simulink model "cgMassInertia"  (R2024a)
settings: configuration reference "autoCodeSILConfigurationParams" (kept outside this file)
undefined symbols (not defined in the file): stepSize_s, vehicleParams
settings Model: Creator=GTAR  LastModifiedBy=jerem
settings ConfigSetRef: SourceName=autoCodeSILConfigurationParams  SourceLocation=Base Workspace

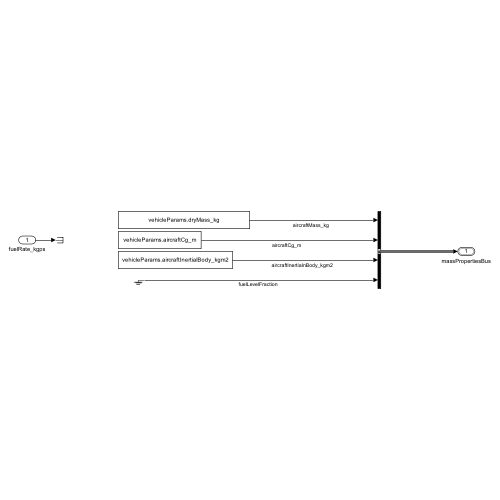
[thumbnail: Simulink's stored preview of the top-level diagram]
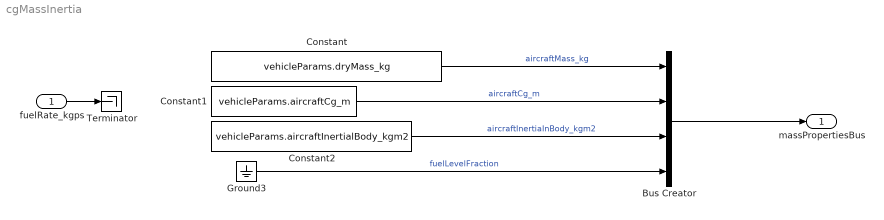
== system cgMassInertia ==
  fuelRate_kgps : Inport
  Bus Creator : BusCreator  Inputs=4  OutDataTypeStr=Bus: MassPropertiesBus  NonVirtualBus=on
  Constant : Constant  Value=vehicleParams.dryMass_kg  SampleTime=stepSize_s
  Constant1 : Constant  Value=vehicleParams.aircraftCg_m  SampleTime=stepSize_s
  Constant2 : Constant  Value=vehicleParams.aircraftInertialBody_kgm2  SampleTime=stepSize_s
  Ground3 : Ground
  Terminator : Terminator
  massPropertiesBus : Outport  OutDataTypeStr=Bus: MassPropertiesBus
  wires:
  Bus Creator/1 -> massPropertiesBus/1
  Constant/1 -> Bus Creator/1  "aircraftMass_kg"
  Constant2/1 -> Bus Creator/3  "aircraftInertiaInBody_kgm2"
  Ground3/1 -> Bus Creator/4  "fuelLevelFraction"
  fuelRate_kgps/1 -> Terminator/1
  Constant1/1 -> Bus Creator/2  "aircraftCg_m"
